simulink model "twobody"  (R2022b)
settings: Solver=ode4  StartTime=0.0  StopTime=simTime  FixedStep=dt  RelTol=1e-3
values from neighbouring files (symbols this model uses):
  initial_position = pq2j2000 ( EarthRadius + EarthOrbitaltitude , 0 , raan , inc , argper )    [main.m]
  initial_velocity = pq2j2000 ( 0 , sqrt ( mu_earth / ( EarthRadius + EarthOrbitaltitude ) ) , raan , inc , argper )    [main.m]
  mu_earth = 398600.4418    [main.m]
  mu_moon = 4911.3    [main.m]
undefined symbols (not defined in the file or in its folder): delv_j2000, lunar_posAtarrival, periods
settings Model: Creator=dongmin  LastModifiedBy=dongmin

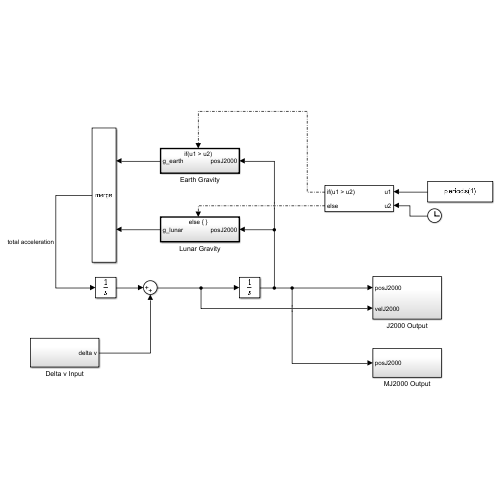
[thumbnail: Simulink's stored preview of the top-level diagram]
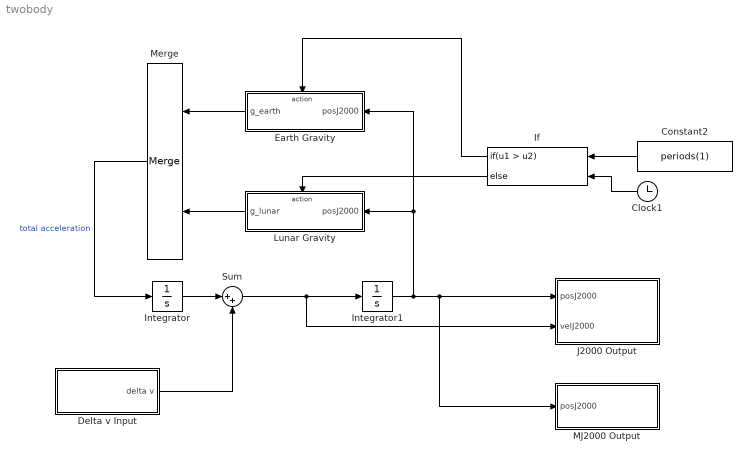
== system twobody ==
  Clock1 : Clock
  Constant2 : Constant  Value=periods(1)
  Delta v Input : Subsystem
  Earth Gravity : Subsystem  TreatAsAtomicUnit=on
  If : If  NumInputs=2  IfExpression=u1 > u2
  Integrator : Integrator  InitialCondition=initial_velocity
  Integrator1 : Integrator  InitialCondition=initial_position
  J2000 Output : Subsystem
  Lunar Gravity : Subsystem  TreatAsAtomicUnit=on
  MJ2000 Output : Subsystem
  Merge : Merge
  Sum : Sum  Inputs=|++
  wires:
  Integrator1/1 -> Earth Gravity/1(posJ2000), Lunar Gravity/1(posJ2000), J2000 Output/1(posJ2000), MJ2000 Output/1(posJ2000)
  Integrator/1 -> Sum/1
  Sum/1 -> J2000 Output/2(velJ2000), Integrator1/1
  Constant2/1 -> If/1
  Earth Gravity/1(g_earth) -> Merge/1
  Lunar Gravity/1(g_lunar) -> Merge/2
  Merge/1 -> Integrator/1  "total acceleration"
  Clock1/1 -> If/2
  If/2 -> Lunar Gravity/Action
  If/1 -> Earth Gravity/Action
  Delta v Input/1(delta v) -> Sum/2

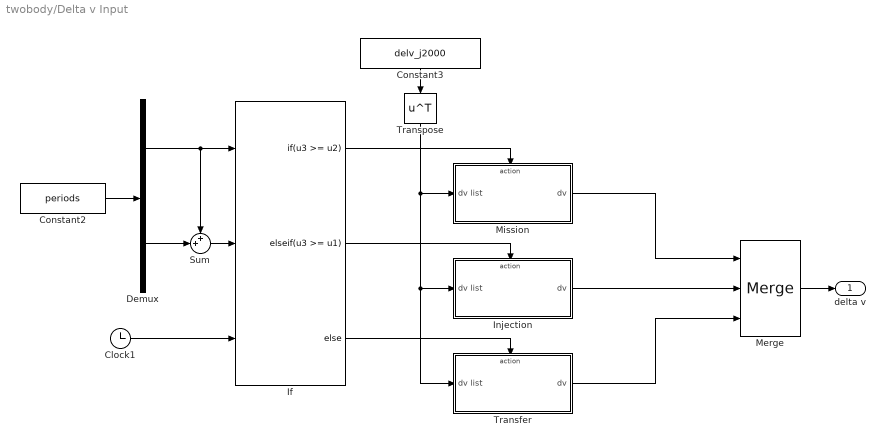
== system twobody/Delta v Input ==
  Clock1 : Clock
  Constant2 : Constant  Value=periods
  Constant3 : Constant  Value=delv_j2000
  Demux : Demux  Outputs=2
  If : If  NumInputs=3  IfExpression=u3 >= u2  ElseIfExpressions=u3 >= u1
  Injection : Subsystem  TreatAsAtomicUnit=on
  Merge : Merge  Inputs=3
  Mission : Subsystem  TreatAsAtomicUnit=on
  Sum : Sum  Inputs=++|
  Transfer : Subsystem  TreatAsAtomicUnit=on
  Transpose : Math  Operator=transpose
  delta v : Outport
  wires:
  Clock1/1 -> If/3
  Constant2/1 -> Demux/1
  Demux/1 -> Sum/1, If/1
  Demux/2 -> Sum/2
  Sum/1 -> If/2
  If/3 -> Transfer/Action
  If/2 -> Injection/Action
  If/1 -> Mission/Action
  Mission/1(dv) -> Merge/1
  Merge/1 -> delta v/1
  Constant3/1 -> Transpose/1
  Injection/1(dv) -> Merge/2
  Transfer/1(dv) -> Merge/3
  Transpose/1 -> Transfer/1(dv list), Injection/1(dv list), Mission/1(dv list)

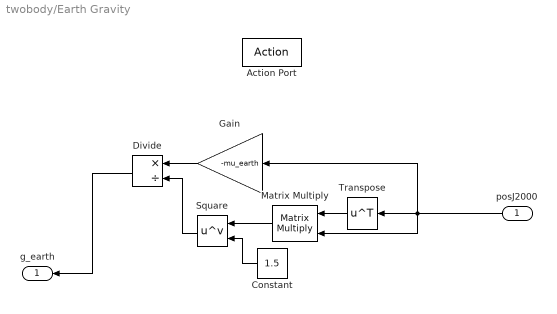
== system twobody/Earth Gravity ==
  posJ2000 : Inport
  Action Port : ActionPort  ActionPortLabel=if(u1 > u2)
  Constant : Constant  Value=1.5
  Divide : Product  Inputs=*/
  Gain : Gain  Gain=-mu_earth
  Matrix Multiply : Product  Multiplication=Matrix(*)
  Square : Math  Operator=pow
  Transpose : Math  Operator=transpose
  g_earth : Outport
  wires:
  Divide/1 -> g_earth/1
  Matrix Multiply/1 -> Square/1
  posJ2000/1 -> Transpose/1, Gain/1, Matrix Multiply/2
  Constant/1 -> Square/2
  Square/1 -> Divide/2
  Transpose/1 -> Matrix Multiply/1
  Gain/1 -> Divide/1

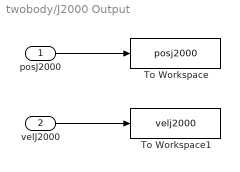
== system twobody/J2000 Output ==
  posJ2000 : Inport
  velJ2000 : Inport  Port=2
  To Workspace : ToWorkspace  VariableName=posj2000  SaveFormat=Timeseries  SampleTime=-1
  To Workspace1 : ToWorkspace  VariableName=velj2000  SaveFormat=Timeseries  SampleTime=-1
  wires:
  velJ2000/1 -> To Workspace1/1
  posJ2000/1 -> To Workspace/1

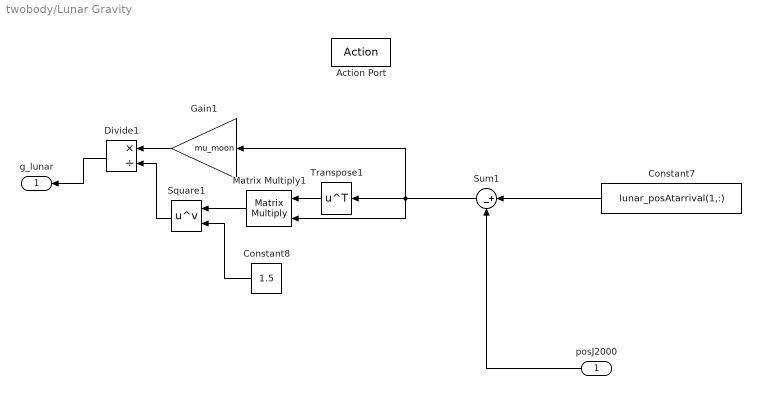
== system twobody/Lunar Gravity ==
  posJ2000 : Inport
  Action Port : ActionPort  ActionPortLabel=else
  Constant7 : Constant  Value=lunar_posAtarrival(1,:)
  Constant8 : Constant  Value=1.5
  Divide1 : Product  Inputs=*/
  Gain1 : Gain  Gain=mu_moon
  Matrix Multiply1 : Product  Multiplication=Matrix(*)
  Square1 : Math  Operator=pow
  Sum1 : Sum  Inputs=|+-
  Transpose1 : Math  Operator=transpose
  g_lunar : Outport
  wires:
  Gain1/1 -> Divide1/1
  Constant8/1 -> Square1/2
  Transpose1/1 -> Matrix Multiply1/1
  Matrix Multiply1/1 -> Square1/1
  posJ2000/1 -> Sum1/2
  Divide1/1 -> g_lunar/1
  Square1/1 -> Divide1/2
  Sum1/1 -> Gain1/1, Matrix Multiply1/2, Transpose1/1
  Constant7/1 -> Sum1/1

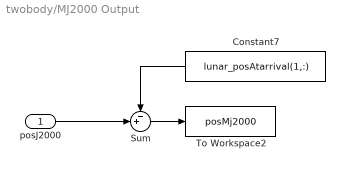
== system twobody/MJ2000 Output ==
  posJ2000 : Inport
  Constant7 : Constant  Value=lunar_posAtarrival(1,:)
  Sum : Sum  Inputs=-+|
  To Workspace2 : ToWorkspace  VariableName=posMj2000  SaveFormat=Timeseries  SampleTime=-1
  wires:
  Constant7/1 -> Sum/1
  posJ2000/1 -> Sum/2
  Sum/1 -> To Workspace2/1

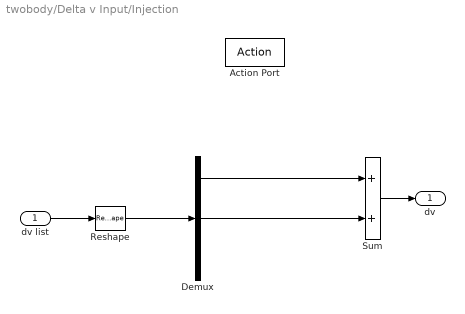
== system twobody/Delta v Input/Injection ==
  dv list : Inport
  Action Port : ActionPort  ActionPortLabel=elseif(u3 >= u1)
  Demux : Demux  Outputs=3
  Reshape : Reshape
  Sum : Sum
  dv : Outport
  wires:
  dv list/1 -> Reshape/1
  Demux/2 -> Sum/2
  Reshape/1 -> Demux/1
  Demux/1 -> Sum/1
  Sum/1 -> dv/1

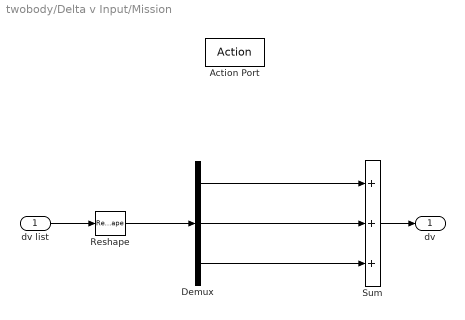
== system twobody/Delta v Input/Mission ==
  dv list : Inport
  Action Port : ActionPort  ActionPortLabel=if(u3 >= u2)
  Demux : Demux  Outputs=3
  Reshape : Reshape
  Sum : Sum  Inputs=+++
  dv : Outport
  wires:
  Sum/1 -> dv/1
  Reshape/1 -> Demux/1
  Demux/1 -> Sum/1
  Demux/2 -> Sum/2
  Demux/3 -> Sum/3
  dv list/1 -> Reshape/1

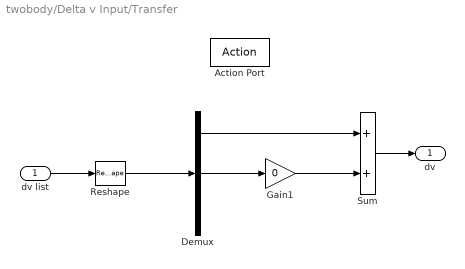
== system twobody/Delta v Input/Transfer ==
  dv list : Inport
  Action Port : ActionPort  ActionPortLabel=else
  Demux : Demux  Outputs=3
  Gain1 : Gain  Gain=0
  Reshape : Reshape
  Sum : Sum
  dv : Outport
  wires:
  dv list/1 -> Reshape/1
  Demux/2 -> Gain1/1
  Reshape/1 -> Demux/1
  Demux/1 -> Sum/1
  Sum/1 -> dv/1
  Gain1/1 -> Sum/2
